simulink model "Ctrl_For_HRV_20260625"  (R2024b)
settings: Solver=ode4  StartTime=0.0  StopTime=22  FixedStep=0.02  RelTol=1e-3
InitFcn:
  | Parameter;
undefined symbols (not defined in the file or in its folder): CCI_DUI_AngleRate_Controller, CCI_DUI_FlowAngle_Controller, fhan, h_alpha, h_beta, h_miu, h_p, h_q, h_r, PNG_2026_6_23, r_alpha, r_beta, r_miu, r_p, r_q, r_r, xishu, xishu_D_0, xishu_L_0, xishu_l_0, xishu_m_0, xishu_n_0, xishu_Y_0
libraries: simulink x60
(part 4 of 8)

== system Ctrl_For_HRV_20260625/Vehicle_2/Error_Model/TD_alpha3 ==
  note: z12
  note: z11
  e_wd_3 : Inport
  Add2 : Sum  Inputs=+-
  Constant : Constant  Value=r_alpha
  Constant1 : Constant  Value=h_alpha
  Integrator : Integrator
  Integrator1 : Integrator
  MATLAB Fcn1 : MATLABFcn  MATLABFcn=fhan(u(1),u(2),u(3),u(4))
  Mux : Mux
  dot_e_wd_3 : Outport  VectorParamsAs1DForOutWhenUnconnected=off
  wires:
  e_wd_3/1 -> Add2/2
  Add2/1 -> Mux/1
  Constant1/1 -> Mux/4
  Constant/1 -> Mux/3
  Mux/1 -> MATLAB Fcn1/1
  MATLAB Fcn1/1 -> Integrator/1
  Integrator1/1 -> Add2/1
  Integrator/1 -> Mux/2, dot_e_wd_3/1, Integrator1/1

== system Ctrl_For_HRV_20260625/Vehicle_2/FlowAngle_Controller_v2/TD_alpha ==
  note: z12
  note: z11
  alpha_d : Inport
  Add2 : Sum  Inputs=+-
  Constant : Constant  Value=r_alpha
  Constant1 : Constant  Value=h_alpha
  Integrator : Integrator
  Integrator1 : Integrator
  MATLAB Fcn1 : MATLABFcn  MATLABFcn=fhan(u(1),u(2),u(3),u(4))
  Mux : Mux
  Scope : Scope
  alpha_c : Outport  VectorParamsAs1DForOutWhenUnconnected=off
  alpha_c_dot : Outport  Port=2  VectorParamsAs1DForOutWhenUnconnected=off
  wires:
  alpha_d/1 -> Add2/2
  Add2/1 -> Mux/1
  Constant1/1 -> Mux/4
  Constant/1 -> Mux/3
  Mux/1 -> MATLAB Fcn1/1
  MATLAB Fcn1/1 -> Integrator/1
  Integrator1/1 -> alpha_c/1, Scope/1, Add2/1
  Integrator/1 -> Mux/2, alpha_c_dot/1, Integrator1/1

== system Ctrl_For_HRV_20260625/Vehicle_2/FlowAngle_Controller_v2/TD_alpha2 ==
  alpha_d : Inport
  Gain17 : Gain  Gain=1.2
  Integrator : Integrator
  Sum : Sum  Inputs=|+-
  alpha_c : Outport
  alpha_c_dot : Outport  Port=2
  wires:
  alpha_d/1 -> Sum/1
  Sum/1 -> Gain17/1
  Integrator/1 -> Sum/2, alpha_c/1
  Gain17/1 -> Integrator/1, alpha_c_dot/1

== system Ctrl_For_HRV_20260625/Vehicle_2/FlowAngle_Controller_v2/TD_alpha3 ==
  note: z12
  note: z11
  dot_beta_c : Inport
  Add2 : Sum  Inputs=+-
  Constant : Constant  Value=r_alpha
  Constant1 : Constant  Value=h_alpha
  Integrator : Integrator
  Integrator1 : Integrator
  MATLAB Fcn1 : MATLABFcn  MATLABFcn=fhan(u(1),u(2),u(3),u(4))
  Mux : Mux
  ddot_beta_c : Outport  VectorParamsAs1DForOutWhenUnconnected=off
  wires:
  dot_beta_c/1 -> Add2/2
  Add2/1 -> Mux/1
  Constant1/1 -> Mux/4
  Constant/1 -> Mux/3
  Mux/1 -> MATLAB Fcn1/1
  MATLAB Fcn1/1 -> Integrator/1
  Integrator1/1 -> Add2/1
  Integrator/1 -> Mux/2, ddot_beta_c/1, Integrator1/1

== system Ctrl_For_HRV_20260625/Vehicle_2/FlowAngle_Controller_v2/TD_alpha4 ==
  note: z12
  note: z11
  dot_miu_c : Inport
  Add2 : Sum  Inputs=+-
  Constant : Constant  Value=r_alpha
  Constant1 : Constant  Value=h_alpha
  Integrator : Integrator
  Integrator1 : Integrator
  MATLAB Fcn1 : MATLABFcn  MATLABFcn=fhan(u(1),u(2),u(3),u(4))
  Mux : Mux
  ddot_miu_c : Outport  VectorParamsAs1DForOutWhenUnconnected=off
  wires:
  dot_miu_c/1 -> Add2/2
  Add2/1 -> Mux/1
  Constant1/1 -> Mux/4
  Constant/1 -> Mux/3
  Mux/1 -> MATLAB Fcn1/1
  MATLAB Fcn1/1 -> Integrator/1
  Integrator1/1 -> Add2/1
  Integrator/1 -> Mux/2, ddot_miu_c/1, Integrator1/1

== system Ctrl_For_HRV_20260625/Vehicle_2/FlowAngle_Controller_v2/TD_beta ==
  note: z12
  note: z11
  beta_d : Inport
  Add2 : Sum  Inputs=+-
  Constant : Constant  Value=r_beta
  Constant1 : Constant  Value=h_beta
  Integrator : Integrator
  Integrator1 : Integrator
  MATLAB Fcn1 : MATLABFcn  MATLABFcn=fhan(u(1),u(2),u(3),u(4))
  Mux : Mux
  beta_c : Outport  VectorParamsAs1DForOutWhenUnconnected=off
  beta_c_dot : Outport  Port=2  VectorParamsAs1DForOutWhenUnconnected=off
  wires:
  beta_d/1 -> Add2/2
  Add2/1 -> Mux/1
  Constant1/1 -> Mux/4
  Constant/1 -> Mux/3
  Mux/1 -> MATLAB Fcn1/1
  MATLAB Fcn1/1 -> Integrator/1
  Integrator1/1 -> beta_c/1, Add2/1
  Integrator/1 -> Mux/2, beta_c_dot/1, Integrator1/1

== system Ctrl_For_HRV_20260625/Vehicle_2/FlowAngle_Controller_v2/TD_beta1 ==
  miu_d : Inport
  Gain17 : Gain  Gain=0.8
  Integrator : Integrator
  Sum : Sum  Inputs=|+-
  miu_c : Outport
  miu_c_dot : Outport  Port=2
  wires:
  miu_d/1 -> Sum/1
  Sum/1 -> Gain17/1
  Integrator/1 -> Sum/2, miu_c/1
  Gain17/1 -> Integrator/1, miu_c_dot/1

== system Ctrl_For_HRV_20260625/Vehicle_2/FlowAngle_Controller_v2/TD_beta2 ==
  beta_d : Inport
  Gain17 : Gain  Gain=1.2
  Integrator : Integrator
  Sum : Sum  Inputs=|+-
  beta_c : Outport
  beta_c_dot : Outport  Port=2
  wires:
  Gain17/1 -> beta_c_dot/1, Integrator/1
  Integrator/1 -> beta_c/1, Sum/2
  Sum/1 -> Gain17/1
  beta_d/1 -> Sum/1

== system Ctrl_For_HRV_20260625/Vehicle_2/FlowAngle_Controller_v2/TD_dotalpha1 ==
  note: z12
  note: z11
  dot_alpha_c : Inport
  Add2 : Sum  Inputs=+-
  Constant : Constant  Value=r_alpha
  Constant1 : Constant  Value=h_alpha
  Integrator : Integrator
  Integrator1 : Integrator
  MATLAB Fcn1 : MATLABFcn  MATLABFcn=fhan(u(1),u(2),u(3),u(4))
  Mux : Mux
  ddot_alpha_c : Outport  VectorParamsAs1DForOutWhenUnconnected=off
  wires:
  dot_alpha_c/1 -> Add2/2
  Add2/1 -> Mux/1
  Constant1/1 -> Mux/4
  Constant/1 -> Mux/3
  Mux/1 -> MATLAB Fcn1/1
  MATLAB Fcn1/1 -> Integrator/1
  Integrator1/1 -> Add2/1
  Integrator/1 -> Mux/2, ddot_alpha_c/1, Integrator1/1

== system Ctrl_For_HRV_20260625/Vehicle_2/FlowAngle_Controller_v2/TD_miu ==
  note: z12
  note: z11
  miu_d : Inport
  Add2 : Sum  Inputs=+-
  Constant : Constant  Value=r_miu
  Constant1 : Constant  Value=h_miu
  Integrator : Integrator
  Integrator1 : Integrator
  MATLAB Fcn1 : MATLABFcn  MATLABFcn=fhan(u(1),u(2),u(3),u(4))
  Mux : Mux
  miu_c : Outport  VectorParamsAs1DForOutWhenUnconnected=off
  miu_c_dot : Outport  Port=2  VectorParamsAs1DForOutWhenUnconnected=off
  wires:
  miu_d/1 -> Add2/2
  Add2/1 -> Mux/1
  Constant1/1 -> Mux/4
  Constant/1 -> Mux/3
  Mux/1 -> MATLAB Fcn1/1
  MATLAB Fcn1/1 -> Integrator/1
  Integrator1/1 -> miu_c/1, Add2/1
  Integrator/1 -> Mux/2, miu_c_dot/1, Integrator1/1

== system Ctrl_For_HRV_20260625/Vehicle_2/HRV_Model_v2/Aerodynamic Parameter perturbation ==
  Band-Limited White Noise : simulink/Sources/Band-Limited White Noise  Cov=1e-6  Ts=2  seed=101
  Band-Limited White Noise1 : simulink/Sources/Band-Limited White Noise  Cov=1e-6  Ts=2  seed=102
  Band-Limited White Noise10 : simulink/Sources/Band-Limited White Noise  Cov=1e-10  Ts=2  seed=103
  Band-Limited White Noise11 : simulink/Sources/Band-Limited White Noise  Cov=1e-10  Ts=2  seed=104
  Band-Limited White Noise12 : simulink/Sources/Band-Limited White Noise  Cov=1e-10  Ts=2  seed=105
  Band-Limited White Noise13 : simulink/Sources/Band-Limited White Noise  Cov=1e-10  Ts=2  seed=106
  Band-Limited White Noise4 : simulink/Sources/Band-Limited White Noise  Cov=1e-6  Ts=2  seed=107
  Band-Limited White Noise5 : simulink/Sources/Band-Limited White Noise  Cov=1e-6  Ts=2  seed=108
  Band-Limited White Noise6 : simulink/Sources/Band-Limited White Noise  Cov=1e-6  Ts=2  seed=109
  Band-Limited White Noise7 : simulink/Sources/Band-Limited White Noise  Cov=1e-6  Ts=2  seed=110
  Band-Limited White Noise8 : simulink/Sources/Band-Limited White Noise  Cov=1e-10  Ts=2  seed=111
  Band-Limited White Noise9 : simulink/Sources/Band-Limited White Noise  Cov=1e-10  Ts=2  seed=112
  Demux : Demux  Outputs=12
  Integrator : Integrator  InitialCondition=[xishu_L_0,xishu_D_0,xishu_Y_0,xishu_l_0,xishu_m_0,xishu_n_0,0,0,0,0,0,0]
  MATLAB Function : MATLAB Function  TreatAsAtomicUnit=on
  Mux : Mux  Inputs=12
  Scope{1..6} (6 alike) : Scope
  To Workspace : ToWorkspace  VariableName=C_L_d_v2  SampleTime=-1
      settings: Save2DSignal=2-D array (concatenate along first dimension)
  To Workspace1 : ToWorkspace  VariableName=C_D_d_v2  SampleTime=-1
      settings: Save2DSignal=2-D array (concatenate along first dimension)
  To Workspace2 : ToWorkspace  VariableName=C_Y_d_v2  SampleTime=-1
      settings: Save2DSignal=2-D array (concatenate along first dimension)
  To Workspace3 : ToWorkspace  VariableName=C_l_d_v2  SampleTime=-1
      settings: Save2DSignal=2-D array (concatenate along first dimension)
  To Workspace4 : ToWorkspace  VariableName=C_m_d_v2  SampleTime=-1
      settings: Save2DSignal=2-D array (concatenate along first dimension)
  To Workspace5 : ToWorkspace  VariableName=C_n_d_v2  SampleTime=-1
      settings: Save2DSignal=2-D array (concatenate along first dimension)
  tag scope: C_D_d_v2=global, C_L_d_v2=global, C_Y_d_v2=global, C_l_d_v2=global, C_m_d_v2=global, C_n_d_v2=global
  wires:
  [C_n_d_v2] -> To Workspace5/1
  [C_m_d_v2] -> To Workspace4/1
  [C_l_d_v2] -> To Workspace3/1
  [C_Y_d_v2] -> To Workspace2/1
  [C_L_d_v2] -> To Workspace/1
  [C_D_d_v2] -> To Workspace1/1
  [C_D_d_v2] -> Scope1/1
  [C_L_d_v2] -> Scope6/1
  [C_l_d_v2] -> Scope3/1
  [C_n_d_v2] -> Scope5/1
  [C_m_d_v2] -> Scope4/1
  [C_Y_d_v2] -> Scope2/1
  Demux/6 -> [C_n_d_v2]
  Demux/5 -> [C_m_d_v2]
  Demux/4 -> [C_l_d_v2]
  Demux/3 -> [C_Y_d_v2]
  Demux/2 -> [C_D_d_v2]
  Demux/1 -> [C_L_d_v2]
  Integrator/1 -> MATLAB Function/1(state), Demux/1
  MATLAB Function/1(dot_state) -> Integrator/1
  Band-Limited White Noise13/1 -> Mux/12
  Band-Limited White Noise12/1 -> Mux/11
  Band-Limited White Noise11/1 -> Mux/10
  Band-Limited White Noise10/1 -> Mux/9
  Band-Limited White Noise9/1 -> Mux/8
  Band-Limited White Noise8/1 -> Mux/7
  Band-Limited White Noise7/1 -> Mux/6
  Band-Limited White Noise6/1 -> Mux/5
  Band-Limited White Noise4/1 -> Mux/3
  Band-Limited White Noise5/1 -> Mux/4
  Band-Limited White Noise1/1 -> Mux/2
  Band-Limited White Noise/1 -> Mux/1
  Mux/1 -> MATLAB Function/2(u)

== system Ctrl_For_HRV_20260625/Vehicle_3/AngleRate_Controller_v3/TD_p ==
  note: z12
  note: z11
  p_d : Inport
  Add2 : Sum  Inputs=+-
  Constant : Constant  Value=r_p
  Constant1 : Constant  Value=h_p
  Integrator : Integrator
  Integrator1 : Integrator
  MATLAB Fcn1 : MATLABFcn  MATLABFcn=fhan(u(1),u(2),u(3),u(4))
  Mux : Mux
  p_c : Outport  VectorParamsAs1DForOutWhenUnconnected=off
  p_c_dot : Outport  Port=2  VectorParamsAs1DForOutWhenUnconnected=off
  wires:
  p_d/1 -> Add2/2
  Add2/1 -> Mux/1
  Constant1/1 -> Mux/4
  Constant/1 -> Mux/3
  Mux/1 -> MATLAB Fcn1/1
  MATLAB Fcn1/1 -> Integrator/1
  Integrator1/1 -> p_c/1, Add2/1
  Integrator/1 -> Mux/2, p_c_dot/1, Integrator1/1

== system Ctrl_For_HRV_20260625/Vehicle_3/AngleRate_Controller_v3/TD_q ==
  note: z12
  note: z11
  q_d : Inport
  Add2 : Sum  Inputs=+-
  Constant : Constant  Value=r_q
  Constant1 : Constant  Value=h_q
  Integrator : Integrator
  Integrator1 : Integrator
  MATLAB Fcn1 : MATLABFcn  MATLABFcn=fhan(u(1),u(2),u(3),u(4))
  Mux : Mux
  q_c : Outport  VectorParamsAs1DForOutWhenUnconnected=off
  q_c_dot : Outport  Port=2  VectorParamsAs1DForOutWhenUnconnected=off
  wires:
  q_d/1 -> Add2/2
  Add2/1 -> Mux/1
  Constant1/1 -> Mux/4
  Constant/1 -> Mux/3
  Mux/1 -> MATLAB Fcn1/1
  MATLAB Fcn1/1 -> Integrator/1
  Integrator1/1 -> q_c/1, Add2/1
  Integrator/1 -> Mux/2, q_c_dot/1, Integrator1/1

== system Ctrl_For_HRV_20260625/Vehicle_3/AngleRate_Controller_v3/TD_r ==
  note: z12
  note: z11
  r_d : Inport
  Add2 : Sum  Inputs=+-
  Constant : Constant  Value=r_r
  Constant1 : Constant  Value=h_r
  Integrator : Integrator
  Integrator1 : Integrator
  MATLAB Fcn1 : MATLABFcn  MATLABFcn=fhan(u(1),u(2),u(3),u(4))
  Mux : Mux
  r_c : Outport  VectorParamsAs1DForOutWhenUnconnected=off
  r_c_dot : Outport  Port=2  VectorParamsAs1DForOutWhenUnconnected=off
  wires:
  r_d/1 -> Add2/2
  Add2/1 -> Mux/1
  Constant1/1 -> Mux/4
  Constant/1 -> Mux/3
  Mux/1 -> MATLAB Fcn1/1
  MATLAB Fcn1/1 -> Integrator/1
  Integrator1/1 -> r_c/1, Add2/1
  Integrator/1 -> Mux/2, r_c_dot/1, Integrator1/1

== system Ctrl_For_HRV_20260625/Vehicle_3/Error_Model/TD_alpha1 ==
  note: z12
  note: z11
  e_wd_1 : Inport
  Add2 : Sum  Inputs=+-
  Constant : Constant  Value=r_alpha
  Constant1 : Constant  Value=h_alpha
  Integrator : Integrator
  Integrator1 : Integrator
  MATLAB Fcn1 : MATLABFcn  MATLABFcn=fhan(u(1),u(2),u(3),u(4))
  Mux : Mux
  dot_e_wd_1 : Outport  VectorParamsAs1DForOutWhenUnconnected=off
  wires:
  e_wd_1/1 -> Add2/2
  Add2/1 -> Mux/1
  Constant1/1 -> Mux/4
  Constant/1 -> Mux/3
  Mux/1 -> MATLAB Fcn1/1
  MATLAB Fcn1/1 -> Integrator/1
  Integrator1/1 -> Add2/1
  Integrator/1 -> Mux/2, dot_e_wd_1/1, Integrator1/1

== system Ctrl_For_HRV_20260625/Vehicle_3/Error_Model/TD_alpha2 ==
  note: z11
  note: z12
  e_wd_2 : Inport
  Add2 : Sum  Inputs=+-
  Constant : Constant  Value=r_alpha
  Constant1 : Constant  Value=h_alpha
  Integrator : Integrator
  Integrator1 : Integrator
  MATLAB Fcn1 : MATLABFcn  MATLABFcn=fhan(u(1),u(2),u(3),u(4))
  Mux : Mux
  dot_e_wd_2 : Outport  VectorParamsAs1DForOutWhenUnconnected=off
  wires:
  Integrator/1 -> Integrator1/1, dot_e_wd_2/1, Mux/2
  Integrator1/1 -> Add2/1
  MATLAB Fcn1/1 -> Integrator/1
  Mux/1 -> MATLAB Fcn1/1
  Constant/1 -> Mux/3
  Constant1/1 -> Mux/4
  Add2/1 -> Mux/1
  e_wd_2/1 -> Add2/2

== system Ctrl_For_HRV_20260625/Vehicle_3/Error_Model/TD_alpha3 ==
  note: z12
  note: z11
  e_wd_3 : Inport
  Add2 : Sum  Inputs=+-
  Constant : Constant  Value=r_alpha
  Constant1 : Constant  Value=h_alpha
  Integrator : Integrator
  Integrator1 : Integrator
  MATLAB Fcn1 : MATLABFcn  MATLABFcn=fhan(u(1),u(2),u(3),u(4))
  Mux : Mux
  dot_e_wd_3 : Outport  VectorParamsAs1DForOutWhenUnconnected=off
  wires:
  e_wd_3/1 -> Add2/2
  Add2/1 -> Mux/1
  Constant1/1 -> Mux/4
  Constant/1 -> Mux/3
  Mux/1 -> MATLAB Fcn1/1
  MATLAB Fcn1/1 -> Integrator/1
  Integrator1/1 -> Add2/1
  Integrator/1 -> Mux/2, dot_e_wd_3/1, Integrator1/1

== system Ctrl_For_HRV_20260625/Vehicle_3/FlowAngle_Controller_v3/TD_alpha ==
  note: z12
  note: z11
  alpha_d : Inport
  Add2 : Sum  Inputs=+-
  Constant : Constant  Value=r_alpha
  Constant1 : Constant  Value=h_alpha
  Integrator : Integrator
  Integrator1 : Integrator
  MATLAB Fcn1 : MATLABFcn  MATLABFcn=fhan(u(1),u(2),u(3),u(4))
  Mux : Mux
  Scope : Scope
  alpha_c : Outport  VectorParamsAs1DForOutWhenUnconnected=off
  alpha_c_dot : Outport  Port=2  VectorParamsAs1DForOutWhenUnconnected=off
  wires:
  alpha_d/1 -> Add2/2
  Add2/1 -> Mux/1
  Constant1/1 -> Mux/4
  Constant/1 -> Mux/3
  Mux/1 -> MATLAB Fcn1/1
  MATLAB Fcn1/1 -> Integrator/1
  Integrator1/1 -> alpha_c/1, Scope/1, Add2/1
  Integrator/1 -> Mux/2, alpha_c_dot/1, Integrator1/1

== system Ctrl_For_HRV_20260625/Vehicle_3/FlowAngle_Controller_v3/TD_alpha2 ==
  alpha_d : Inport
  Gain17 : Gain  Gain=1.2
  Integrator : Integrator
  Sum : Sum  Inputs=|+-
  alpha_c : Outport
  alpha_c_dot : Outport  Port=2
  wires:
  alpha_d/1 -> Sum/1
  Sum/1 -> Gain17/1
  Integrator/1 -> Sum/2, alpha_c/1
  Gain17/1 -> Integrator/1, alpha_c_dot/1

== system Ctrl_For_HRV_20260625/Vehicle_3/FlowAngle_Controller_v3/TD_alpha3 ==
  note: z12
  note: z11
  dot_beta_c : Inport
  Add2 : Sum  Inputs=+-
  Constant : Constant  Value=r_alpha
  Constant1 : Constant  Value=h_alpha
  Integrator : Integrator
  Integrator1 : Integrator
  MATLAB Fcn1 : MATLABFcn  MATLABFcn=fhan(u(1),u(2),u(3),u(4))
  Mux : Mux
  ddot_beta_c : Outport  VectorParamsAs1DForOutWhenUnconnected=off
  wires:
  dot_beta_c/1 -> Add2/2
  Add2/1 -> Mux/1
  Constant1/1 -> Mux/4
  Constant/1 -> Mux/3
  Mux/1 -> MATLAB Fcn1/1
  MATLAB Fcn1/1 -> Integrator/1
  Integrator1/1 -> Add2/1
  Integrator/1 -> Mux/2, ddot_beta_c/1, Integrator1/1

== system Ctrl_For_HRV_20260625/Vehicle_3/FlowAngle_Controller_v3/TD_alpha4 ==
  note: z12
  note: z11
  dot_miu_c : Inport
  Add2 : Sum  Inputs=+-
  Constant : Constant  Value=r_alpha
  Constant1 : Constant  Value=h_alpha
  Integrator : Integrator
  Integrator1 : Integrator
  MATLAB Fcn1 : MATLABFcn  MATLABFcn=fhan(u(1),u(2),u(3),u(4))
  Mux : Mux
  ddot_miu_c : Outport  VectorParamsAs1DForOutWhenUnconnected=off
  wires:
  dot_miu_c/1 -> Add2/2
  Add2/1 -> Mux/1
  Constant1/1 -> Mux/4
  Constant/1 -> Mux/3
  Mux/1 -> MATLAB Fcn1/1
  MATLAB Fcn1/1 -> Integrator/1
  Integrator1/1 -> Add2/1
  Integrator/1 -> Mux/2, ddot_miu_c/1, Integrator1/1

== system Ctrl_For_HRV_20260625/Vehicle_3/FlowAngle_Controller_v3/TD_beta ==
  note: z12
  note: z11
  beta_d : Inport
  Add2 : Sum  Inputs=+-
  Constant : Constant  Value=r_beta
  Constant1 : Constant  Value=h_beta
  Integrator : Integrator
  Integrator1 : Integrator
  MATLAB Fcn1 : MATLABFcn  MATLABFcn=fhan(u(1),u(2),u(3),u(4))
  Mux : Mux
  beta_c : Outport  VectorParamsAs1DForOutWhenUnconnected=off
  beta_c_dot : Outport  Port=2  VectorParamsAs1DForOutWhenUnconnected=off
  wires:
  beta_d/1 -> Add2/2
  Add2/1 -> Mux/1
  Constant1/1 -> Mux/4
  Constant/1 -> Mux/3
  Mux/1 -> MATLAB Fcn1/1
  MATLAB Fcn1/1 -> Integrator/1
  Integrator1/1 -> beta_c/1, Add2/1
  Integrator/1 -> Mux/2, beta_c_dot/1, Integrator1/1

== system Ctrl_For_HRV_20260625/Vehicle_3/FlowAngle_Controller_v3/TD_beta1 ==
  miu_d : Inport
  Gain17 : Gain  Gain=0.8
  Integrator : Integrator
  Sum : Sum  Inputs=|+-
  miu_c : Outport
  miu_c_dot : Outport  Port=2
  wires:
  miu_d/1 -> Sum/1
  Sum/1 -> Gain17/1
  Integrator/1 -> Sum/2, miu_c/1
  Gain17/1 -> Integrator/1, miu_c_dot/1

== system Ctrl_For_HRV_20260625/Vehicle_3/FlowAngle_Controller_v3/TD_beta2 ==
  beta_d : Inport
  Gain17 : Gain  Gain=1.2
  Integrator : Integrator
  Sum : Sum  Inputs=|+-
  beta_c : Outport
  beta_c_dot : Outport  Port=2
  wires:
  Gain17/1 -> beta_c_dot/1, Integrator/1
  Integrator/1 -> beta_c/1, Sum/2
  Sum/1 -> Gain17/1
  beta_d/1 -> Sum/1

== system Ctrl_For_HRV_20260625/Vehicle_3/FlowAngle_Controller_v3/TD_dotalpha1 ==
  note: z12
  note: z11
  dot_alpha_c : Inport
  Add2 : Sum  Inputs=+-
  Constant : Constant  Value=r_alpha
  Constant1 : Constant  Value=h_alpha
  Integrator : Integrator
  Integrator1 : Integrator
  MATLAB Fcn1 : MATLABFcn  MATLABFcn=fhan(u(1),u(2),u(3),u(4))
  Mux : Mux
  ddot_alpha_c : Outport  VectorParamsAs1DForOutWhenUnconnected=off
  wires:
  dot_alpha_c/1 -> Add2/2
  Add2/1 -> Mux/1
  Constant1/1 -> Mux/4
  Constant/1 -> Mux/3
  Mux/1 -> MATLAB Fcn1/1
  MATLAB Fcn1/1 -> Integrator/1
  Integrator1/1 -> Add2/1
  Integrator/1 -> Mux/2, ddot_alpha_c/1, Integrator1/1

== system Ctrl_For_HRV_20260625/Vehicle_3/FlowAngle_Controller_v3/TD_miu ==
  note: z12
  note: z11
  miu_d : Inport
  Add2 : Sum  Inputs=+-
  Constant : Constant  Value=r_miu
  Constant1 : Constant  Value=h_miu
  Integrator : Integrator
  Integrator1 : Integrator
  MATLAB Fcn1 : MATLABFcn  MATLABFcn=fhan(u(1),u(2),u(3),u(4))
  Mux : Mux
  miu_c : Outport  VectorParamsAs1DForOutWhenUnconnected=off
  miu_c_dot : Outport  Port=2  VectorParamsAs1DForOutWhenUnconnected=off
  wires:
  miu_d/1 -> Add2/2
  Add2/1 -> Mux/1
  Constant1/1 -> Mux/4
  Constant/1 -> Mux/3
  Mux/1 -> MATLAB Fcn1/1
  MATLAB Fcn1/1 -> Integrator/1
  Integrator1/1 -> miu_c/1, Add2/1
  Integrator/1 -> Mux/2, miu_c_dot/1, Integrator1/1

== system Ctrl_For_HRV_20260625/Vehicle_3/HRV_Model_v3/Aerodynamic Parameter perturbation ==
  Band-Limited White Noise : simulink/Sources/Band-Limited White Noise  Cov=1e-6  Ts=2  seed=101
  Band-Limited White Noise1 : simulink/Sources/Band-Limited White Noise  Cov=1e-6  Ts=2  seed=102
  Band-Limited White Noise10 : simulink/Sources/Band-Limited White Noise  Cov=1e-10  Ts=2  seed=103
  Band-Limited White Noise11 : simulink/Sources/Band-Limited White Noise  Cov=1e-10  Ts=2  seed=104
  Band-Limited White Noise12 : simulink/Sources/Band-Limited White Noise  Cov=1e-10  Ts=2  seed=105
  Band-Limited White Noise13 : simulink/Sources/Band-Limited White Noise  Cov=1e-10  Ts=2  seed=106
  Band-Limited White Noise4 : simulink/Sources/Band-Limited White Noise  Cov=1e-6  Ts=2  seed=107
  Band-Limited White Noise5 : simulink/Sources/Band-Limited White Noise  Cov=1e-6  Ts=2  seed=108
  Band-Limited White Noise6 : simulink/Sources/Band-Limited White Noise  Cov=1e-6  Ts=2  seed=109
  Band-Limited White Noise7 : simulink/Sources/Band-Limited White Noise  Cov=1e-6  Ts=2  seed=110
  Band-Limited White Noise8 : simulink/Sources/Band-Limited White Noise  Cov=1e-10  Ts=2  seed=111
  Band-Limited White Noise9 : simulink/Sources/Band-Limited White Noise  Cov=1e-10  Ts=2  seed=112
  Demux : Demux  Outputs=12
  Integrator : Integrator  InitialCondition=[xishu_L_0,xishu_D_0,xishu_Y_0,xishu_l_0,xishu_m_0,xishu_n_0,0,0,0,0,0,0]
  MATLAB Function : MATLAB Function  TreatAsAtomicUnit=on
  Mux : Mux  Inputs=12
  Scope{1..6} (6 alike) : Scope
  To Workspace : ToWorkspace  VariableName=C_L_d_v3  SampleTime=-1
      settings: Save2DSignal=2-D array (concatenate along first dimension)
  To Workspace1 : ToWorkspace  VariableName=C_D_d_v3  SampleTime=-1
      settings: Save2DSignal=2-D array (concatenate along first dimension)
  To Workspace2 : ToWorkspace  VariableName=C_Y_d_v3  SampleTime=-1
      settings: Save2DSignal=2-D array (concatenate along first dimension)
  To Workspace3 : ToWorkspace  VariableName=C_l_d_v3  SampleTime=-1
      settings: Save2DSignal=2-D array (concatenate along first dimension)
  To Workspace4 : ToWorkspace  VariableName=C_m_d_v3  SampleTime=-1
      settings: Save2DSignal=2-D array (concatenate along first dimension)
  To Workspace5 : ToWorkspace  VariableName=C_n_d_v3  SampleTime=-1
      settings: Save2DSignal=2-D array (concatenate along first dimension)
  tag scope: C_D_d_v3=global, C_L_d_v3=global, C_Y_d_v3=global, C_l_d_v3=global, C_m_d_v3=global, C_n_d_v3=global
  wires:
  [C_n_d_v3] -> To Workspace5/1
  [C_m_d_v3] -> To Workspace4/1
  [C_l_d_v3] -> To Workspace3/1
  [C_Y_d_v3] -> To Workspace2/1
  [C_L_d_v3] -> To Workspace/1
  [C_D_d_v3] -> To Workspace1/1
  [C_D_d_v3] -> Scope1/1
  [C_L_d_v3] -> Scope6/1
  [C_l_d_v3] -> Scope3/1
  [C_n_d_v3] -> Scope5/1
  [C_m_d_v3] -> Scope4/1
  [C_Y_d_v3] -> Scope2/1
  Demux/6 -> [C_n_d_v3]
  Demux/5 -> [C_m_d_v3]
  Demux/4 -> [C_l_d_v3]
  Demux/3 -> [C_Y_d_v3]
  Demux/2 -> [C_D_d_v3]
  Demux/1 -> [C_L_d_v3]
  Integrator/1 -> MATLAB Function/1(state), Demux/1
  MATLAB Function/1(dot_state) -> Integrator/1
  Band-Limited White Noise13/1 -> Mux/12
  Band-Limited White Noise12/1 -> Mux/11
  Band-Limited White Noise11/1 -> Mux/10
  Band-Limited White Noise10/1 -> Mux/9
  Band-Limited White Noise9/1 -> Mux/8
  Band-Limited White Noise8/1 -> Mux/7
  Band-Limited White Noise7/1 -> Mux/6
  Band-Limited White Noise6/1 -> Mux/5
  Band-Limited White Noise4/1 -> Mux/3
  Band-Limited White Noise5/1 -> Mux/4
  Band-Limited White Noise1/1 -> Mux/2
  Band-Limited White Noise/1 -> Mux/1
  Mux/1 -> MATLAB Function/2(u)

== system Ctrl_For_HRV_20260625/Vehicle_4/AngleRate_Controller_v4/TD_p ==
  note: z12
  note: z11
  p_d : Inport
  Add2 : Sum  Inputs=+-
  Constant : Constant  Value=r_p
  Constant1 : Constant  Value=h_p
  Integrator : Integrator
  Integrator1 : Integrator
  MATLAB Fcn1 : MATLABFcn  MATLABFcn=fhan(u(1),u(2),u(3),u(4))
  Mux : Mux
  p_c : Outport  VectorParamsAs1DForOutWhenUnconnected=off
  p_c_dot : Outport  Port=2  VectorParamsAs1DForOutWhenUnconnected=off
  wires:
  p_d/1 -> Add2/2
  Add2/1 -> Mux/1
  Constant1/1 -> Mux/4
  Constant/1 -> Mux/3
  Mux/1 -> MATLAB Fcn1/1
  MATLAB Fcn1/1 -> Integrator/1
  Integrator1/1 -> p_c/1, Add2/1
  Integrator/1 -> Mux/2, p_c_dot/1, Integrator1/1

== system Ctrl_For_HRV_20260625/Vehicle_4/AngleRate_Controller_v4/TD_q ==
  note: z12
  note: z11
  q_d : Inport
  Add2 : Sum  Inputs=+-
  Constant : Constant  Value=r_q
  Constant1 : Constant  Value=h_q
  Integrator : Integrator
  Integrator1 : Integrator
  MATLAB Fcn1 : MATLABFcn  MATLABFcn=fhan(u(1),u(2),u(3),u(4))
  Mux : Mux
  q_c : Outport  VectorParamsAs1DForOutWhenUnconnected=off
  q_c_dot : Outport  Port=2  VectorParamsAs1DForOutWhenUnconnected=off
  wires:
  q_d/1 -> Add2/2
  Add2/1 -> Mux/1
  Constant1/1 -> Mux/4
  Constant/1 -> Mux/3
  Mux/1 -> MATLAB Fcn1/1
  MATLAB Fcn1/1 -> Integrator/1
  Integrator1/1 -> q_c/1, Add2/1
  Integrator/1 -> Mux/2, q_c_dot/1, Integrator1/1

== system Ctrl_For_HRV_20260625/Vehicle_4/AngleRate_Controller_v4/TD_r ==
  note: z12
  note: z11
  r_d : Inport
  Add2 : Sum  Inputs=+-
  Constant : Constant  Value=r_r
  Constant1 : Constant  Value=h_r
  Integrator : Integrator
  Integrator1 : Integrator
  MATLAB Fcn1 : MATLABFcn  MATLABFcn=fhan(u(1),u(2),u(3),u(4))
  Mux : Mux
  r_c : Outport  VectorParamsAs1DForOutWhenUnconnected=off
  r_c_dot : Outport  Port=2  VectorParamsAs1DForOutWhenUnconnected=off
  wires:
  r_d/1 -> Add2/2
  Add2/1 -> Mux/1
  Constant1/1 -> Mux/4
  Constant/1 -> Mux/3
  Mux/1 -> MATLAB Fcn1/1
  MATLAB Fcn1/1 -> Integrator/1
  Integrator1/1 -> r_c/1, Add2/1
  Integrator/1 -> Mux/2, r_c_dot/1, Integrator1/1

== system Ctrl_For_HRV_20260625/Vehicle_4/Error_Model/TD_alpha1 ==
  note: z12
  note: z11
  e_wd_1 : Inport
  Add2 : Sum  Inputs=+-
  Constant : Constant  Value=r_alpha
  Constant1 : Constant  Value=h_alpha
  Integrator : Integrator
  Integrator1 : Integrator
  MATLAB Fcn1 : MATLABFcn  MATLABFcn=fhan(u(1),u(2),u(3),u(4))
  Mux : Mux
  dot_e_wd_1 : Outport  VectorParamsAs1DForOutWhenUnconnected=off
  wires:
  e_wd_1/1 -> Add2/2
  Add2/1 -> Mux/1
  Constant1/1 -> Mux/4
  Constant/1 -> Mux/3
  Mux/1 -> MATLAB Fcn1/1
  MATLAB Fcn1/1 -> Integrator/1
  Integrator1/1 -> Add2/1
  Integrator/1 -> Mux/2, dot_e_wd_1/1, Integrator1/1

== system Ctrl_For_HRV_20260625/Vehicle_4/Error_Model/TD_alpha2 ==
  note: z11
  note: z12
  e_wd_2 : Inport
  Add2 : Sum  Inputs=+-
  Constant : Constant  Value=r_alpha
  Constant1 : Constant  Value=h_alpha
  Integrator : Integrator
  Integrator1 : Integrator
  MATLAB Fcn1 : MATLABFcn  MATLABFcn=fhan(u(1),u(2),u(3),u(4))
  Mux : Mux
  dot_e_wd_2 : Outport  VectorParamsAs1DForOutWhenUnconnected=off
  wires:
  Integrator/1 -> Integrator1/1, dot_e_wd_2/1, Mux/2
  Integrator1/1 -> Add2/1
  MATLAB Fcn1/1 -> Integrator/1
  Mux/1 -> MATLAB Fcn1/1
  Constant/1 -> Mux/3
  Constant1/1 -> Mux/4
  Add2/1 -> Mux/1
  e_wd_2/1 -> Add2/2

== system Ctrl_For_HRV_20260625/Vehicle_4/Error_Model/TD_alpha3 ==
  note: z12
  note: z11
  e_wd_3 : Inport
  Add2 : Sum  Inputs=+-
  Constant : Constant  Value=r_alpha
  Constant1 : Constant  Value=h_alpha
  Integrator : Integrator
  Integrator1 : Integrator
  MATLAB Fcn1 : MATLABFcn  MATLABFcn=fhan(u(1),u(2),u(3),u(4))
  Mux : Mux
  dot_e_wd_3 : Outport  VectorParamsAs1DForOutWhenUnconnected=off
  wires:
  e_wd_3/1 -> Add2/2
  Add2/1 -> Mux/1
  Constant1/1 -> Mux/4
  Constant/1 -> Mux/3
  Mux/1 -> MATLAB Fcn1/1
  MATLAB Fcn1/1 -> Integrator/1
  Integrator1/1 -> Add2/1
  Integrator/1 -> Mux/2, dot_e_wd_3/1, Integrator1/1

== system Ctrl_For_HRV_20260625/Vehicle_4/FlowAngle_Controller_v4/TD_alpha ==
  note: z12
  note: z11
  alpha_d : Inport
  Add2 : Sum  Inputs=+-
  Constant : Constant  Value=r_alpha
  Constant1 : Constant  Value=h_alpha
  Integrator : Integrator
  Integrator1 : Integrator
  MATLAB Fcn1 : MATLABFcn  MATLABFcn=fhan(u(1),u(2),u(3),u(4))
  Mux : Mux
  Scope : Scope
  alpha_c : Outport  VectorParamsAs1DForOutWhenUnconnected=off
  alpha_c_dot : Outport  Port=2  VectorParamsAs1DForOutWhenUnconnected=off
  wires:
  alpha_d/1 -> Add2/2
  Add2/1 -> Mux/1
  Constant1/1 -> Mux/4
  Constant/1 -> Mux/3
  Mux/1 -> MATLAB Fcn1/1
  MATLAB Fcn1/1 -> Integrator/1
  Integrator1/1 -> alpha_c/1, Scope/1, Add2/1
  Integrator/1 -> Mux/2, alpha_c_dot/1, Integrator1/1

== system Ctrl_For_HRV_20260625/Vehicle_4/FlowAngle_Controller_v4/TD_alpha2 ==
  alpha_d : Inport
  Gain17 : Gain  Gain=1.2
  Integrator : Integrator
  Sum : Sum  Inputs=|+-
  alpha_c : Outport
  alpha_c_dot : Outport  Port=2
  wires:
  alpha_d/1 -> Sum/1
  Sum/1 -> Gain17/1
  Integrator/1 -> Sum/2, alpha_c/1
  Gain17/1 -> Integrator/1, alpha_c_dot/1

== system Ctrl_For_HRV_20260625/Vehicle_4/FlowAngle_Controller_v4/TD_alpha3 ==
  note: z12
  note: z11
  dot_beta_c : Inport
  Add2 : Sum  Inputs=+-
  Constant : Constant  Value=r_alpha
  Constant1 : Constant  Value=h_alpha
  Integrator : Integrator
  Integrator1 : Integrator
  MATLAB Fcn1 : MATLABFcn  MATLABFcn=fhan(u(1),u(2),u(3),u(4))
  Mux : Mux
  ddot_beta_c : Outport  VectorParamsAs1DForOutWhenUnconnected=off
  wires:
  dot_beta_c/1 -> Add2/2
  Add2/1 -> Mux/1
  Constant1/1 -> Mux/4
  Constant/1 -> Mux/3
  Mux/1 -> MATLAB Fcn1/1
  MATLAB Fcn1/1 -> Integrator/1
  Integrator1/1 -> Add2/1
  Integrator/1 -> Mux/2, ddot_beta_c/1, Integrator1/1

== system Ctrl_For_HRV_20260625/Vehicle_4/FlowAngle_Controller_v4/TD_alpha4 ==
  note: z12
  note: z11
  dot_miu_c : Inport
  Add2 : Sum  Inputs=+-
  Constant : Constant  Value=r_alpha
  Constant1 : Constant  Value=h_alpha
  Integrator : Integrator
  Integrator1 : Integrator
  MATLAB Fcn1 : MATLABFcn  MATLABFcn=fhan(u(1),u(2),u(3),u(4))
  Mux : Mux
  ddot_miu_c : Outport  VectorParamsAs1DForOutWhenUnconnected=off
  wires:
  dot_miu_c/1 -> Add2/2
  Add2/1 -> Mux/1
  Constant1/1 -> Mux/4
  Constant/1 -> Mux/3
  Mux/1 -> MATLAB Fcn1/1
  MATLAB Fcn1/1 -> Integrator/1
  Integrator1/1 -> Add2/1
  Integrator/1 -> Mux/2, ddot_miu_c/1, Integrator1/1

== system Ctrl_For_HRV_20260625/Vehicle_4/FlowAngle_Controller_v4/TD_beta ==
  note: z12
  note: z11
  beta_d : Inport
  Add2 : Sum  Inputs=+-
  Constant : Constant  Value=r_beta
  Constant1 : Constant  Value=h_beta
  Integrator : Integrator
  Integrator1 : Integrator
  MATLAB Fcn1 : MATLABFcn  MATLABFcn=fhan(u(1),u(2),u(3),u(4))
  Mux : Mux
  beta_c : Outport  VectorParamsAs1DForOutWhenUnconnected=off
  beta_c_dot : Outport  Port=2  VectorParamsAs1DForOutWhenUnconnected=off
  wires:
  beta_d/1 -> Add2/2
  Add2/1 -> Mux/1
  Constant1/1 -> Mux/4
  Constant/1 -> Mux/3
  Mux/1 -> MATLAB Fcn1/1
  MATLAB Fcn1/1 -> Integrator/1
  Integrator1/1 -> beta_c/1, Add2/1
  Integrator/1 -> Mux/2, beta_c_dot/1, Integrator1/1

== system Ctrl_For_HRV_20260625/Vehicle_4/FlowAngle_Controller_v4/TD_beta1 ==
  miu_d : Inport
  Gain17 : Gain  Gain=0.8
  Integrator : Integrator
  Sum : Sum  Inputs=|+-
  miu_c : Outport
  miu_c_dot : Outport  Port=2
  wires:
  miu_d/1 -> Sum/1
  Sum/1 -> Gain17/1
  Integrator/1 -> Sum/2, miu_c/1
  Gain17/1 -> Integrator/1, miu_c_dot/1

== system Ctrl_For_HRV_20260625/Vehicle_4/FlowAngle_Controller_v4/TD_beta2 ==
  beta_d : Inport
  Gain17 : Gain  Gain=1.2
  Integrator : Integrator
  Sum : Sum  Inputs=|+-
  beta_c : Outport
  beta_c_dot : Outport  Port=2
  wires:
  Gain17/1 -> beta_c_dot/1, Integrator/1
  Integrator/1 -> beta_c/1, Sum/2
  Sum/1 -> Gain17/1
  beta_d/1 -> Sum/1

== system Ctrl_For_HRV_20260625/Vehicle_4/FlowAngle_Controller_v4/TD_dotalpha1 ==
  note: z12
  note: z11
  dot_alpha_c : Inport
  Add2 : Sum  Inputs=+-
  Constant : Constant  Value=r_alpha
  Constant1 : Constant  Value=h_alpha
  Integrator : Integrator
  Integrator1 : Integrator
  MATLAB Fcn1 : MATLABFcn  MATLABFcn=fhan(u(1),u(2),u(3),u(4))
  Mux : Mux
  ddot_alpha_c : Outport  VectorParamsAs1DForOutWhenUnconnected=off
  wires:
  dot_alpha_c/1 -> Add2/2
  Add2/1 -> Mux/1
  Constant1/1 -> Mux/4
  Constant/1 -> Mux/3
  Mux/1 -> MATLAB Fcn1/1
  MATLAB Fcn1/1 -> Integrator/1
  Integrator1/1 -> Add2/1
  Integrator/1 -> Mux/2, ddot_alpha_c/1, Integrator1/1

== system Ctrl_For_HRV_20260625/Vehicle_4/FlowAngle_Controller_v4/TD_miu ==
  note: z12
  note: z11
  miu_d : Inport
  Add2 : Sum  Inputs=+-
  Constant : Constant  Value=r_miu
  Constant1 : Constant  Value=h_miu
  Integrator : Integrator
  Integrator1 : Integrator
  MATLAB Fcn1 : MATLABFcn  MATLABFcn=fhan(u(1),u(2),u(3),u(4))
  Mux : Mux
  miu_c : Outport  VectorParamsAs1DForOutWhenUnconnected=off
  miu_c_dot : Outport  Port=2  VectorParamsAs1DForOutWhenUnconnected=off
  wires:
  miu_d/1 -> Add2/2
  Add2/1 -> Mux/1
  Constant1/1 -> Mux/4
  Constant/1 -> Mux/3
  Mux/1 -> MATLAB Fcn1/1
  MATLAB Fcn1/1 -> Integrator/1
  Integrator1/1 -> miu_c/1, Add2/1
  Integrator/1 -> Mux/2, miu_c_dot/1, Integrator1/1

== system Ctrl_For_HRV_20260625/Vehicle_4/HRV_Model_v4/Aerodynamic Parameter perturbation ==
  Band-Limited White Noise : simulink/Sources/Band-Limited White Noise  Cov=1e-6  Ts=2  seed=101
  Band-Limited White Noise1 : simulink/Sources/Band-Limited White Noise  Cov=1e-6  Ts=2  seed=102
  Band-Limited White Noise10 : simulink/Sources/Band-Limited White Noise  Cov=1e-10  Ts=2  seed=103
  Band-Limited White Noise11 : simulink/Sources/Band-Limited White Noise  Cov=1e-10  Ts=2  seed=104
  Band-Limited White Noise12 : simulink/Sources/Band-Limited White Noise  Cov=1e-10  Ts=2  seed=105
  Band-Limited White Noise13 : simulink/Sources/Band-Limited White Noise  Cov=1e-10  Ts=2  seed=106
  Band-Limited White Noise4 : simulink/Sources/Band-Limited White Noise  Cov=1e-6  Ts=2  seed=107
  Band-Limited White Noise5 : simulink/Sources/Band-Limited White Noise  Cov=1e-6  Ts=2  seed=108
  Band-Limited White Noise6 : simulink/Sources/Band-Limited White Noise  Cov=1e-6  Ts=2  seed=109
  Band-Limited White Noise7 : simulink/Sources/Band-Limited White Noise  Cov=1e-6  Ts=2  seed=110
  Band-Limited White Noise8 : simulink/Sources/Band-Limited White Noise  Cov=1e-10  Ts=2  seed=111
  Band-Limited White Noise9 : simulink/Sources/Band-Limited White Noise  Cov=1e-10  Ts=2  seed=112
  Demux : Demux  Outputs=12
  Integrator : Integrator  InitialCondition=[xishu_L_0,xishu_D_0,xishu_Y_0,xishu_l_0,xishu_m_0,xishu_n_0,0,0,0,0,0,0]
  MATLAB Function : MATLAB Function  TreatAsAtomicUnit=on
  Mux : Mux  Inputs=12
  Scope{1..6} (6 alike) : Scope
  To Workspace : ToWorkspace  VariableName=C_L_d_v4  SampleTime=-1
      settings: Save2DSignal=2-D array (concatenate along first dimension)
  To Workspace1 : ToWorkspace  VariableName=C_D_d_v4  SampleTime=-1
      settings: Save2DSignal=2-D array (concatenate along first dimension)
  To Workspace2 : ToWorkspace  VariableName=C_Y_d_v4  SampleTime=-1
      settings: Save2DSignal=2-D array (concatenate along first dimension)
  To Workspace3 : ToWorkspace  VariableName=C_l_d_v4  SampleTime=-1
      settings: Save2DSignal=2-D array (concatenate along first dimension)
  To Workspace4 : ToWorkspace  VariableName=C_m_d_v4  SampleTime=-1
      settings: Save2DSignal=2-D array (concatenate along first dimension)
  To Workspace5 : ToWorkspace  VariableName=C_n_d_v4  SampleTime=-1
      settings: Save2DSignal=2-D array (concatenate along first dimension)
  tag scope: C_D_d_v4=global, C_L_d_v4=global, C_Y_d_v4=global, C_l_d_v4=global, C_m_d_v4=global, C_n_d_v4=global
  wires:
  [C_n_d_v4] -> To Workspace5/1
  [C_m_d_v4] -> To Workspace4/1
  [C_l_d_v4] -> To Workspace3/1
  [C_Y_d_v4] -> To Workspace2/1
  [C_L_d_v4] -> To Workspace/1
  [C_D_d_v4] -> To Workspace1/1
  [C_D_d_v4] -> Scope1/1
  [C_L_d_v4] -> Scope6/1
  [C_l_d_v4] -> Scope3/1
  [C_n_d_v4] -> Scope5/1
  [C_m_d_v4] -> Scope4/1
  [C_Y_d_v4] -> Scope2/1
  Demux/6 -> [C_n_d_v4]
  Demux/5 -> [C_m_d_v4]
  Demux/4 -> [C_l_d_v4]
  Demux/3 -> [C_Y_d_v4]
  Demux/2 -> [C_D_d_v4]
  Demux/1 -> [C_L_d_v4]
  Integrator/1 -> MATLAB Function/1(state), Demux/1
  MATLAB Function/1(dot_state) -> Integrator/1
  Band-Limited White Noise13/1 -> Mux/12
  Band-Limited White Noise12/1 -> Mux/11
  Band-Limited White Noise11/1 -> Mux/10
  Band-Limited White Noise10/1 -> Mux/9
  Band-Limited White Noise9/1 -> Mux/8
  Band-Limited White Noise8/1 -> Mux/7
  Band-Limited White Noise7/1 -> Mux/6
  Band-Limited White Noise6/1 -> Mux/5
  Band-Limited White Noise4/1 -> Mux/3
  Band-Limited White Noise5/1 -> Mux/4
  Band-Limited White Noise1/1 -> Mux/2
  Band-Limited White Noise/1 -> Mux/1
  Mux/1 -> MATLAB Function/2(u)

== system Ctrl_For_HRV_20260625/Vehicle_5/AngleRate_Controller_v5/TD_p ==
  note: z12
  note: z11
  p_d : Inport
  Add2 : Sum  Inputs=+-
  Constant : Constant  Value=r_p
  Constant1 : Constant  Value=h_p
  Integrator : Integrator
  Integrator1 : Integrator
  MATLAB Fcn1 : MATLABFcn  MATLABFcn=fhan(u(1),u(2),u(3),u(4))
  Mux : Mux
  p_c : Outport  VectorParamsAs1DForOutWhenUnconnected=off
  p_c_dot : Outport  Port=2  VectorParamsAs1DForOutWhenUnconnected=off
  wires:
  p_d/1 -> Add2/2
  Add2/1 -> Mux/1
  Constant1/1 -> Mux/4
  Constant/1 -> Mux/3
  Mux/1 -> MATLAB Fcn1/1
  MATLAB Fcn1/1 -> Integrator/1
  Integrator1/1 -> p_c/1, Add2/1
  Integrator/1 -> Mux/2, p_c_dot/1, Integrator1/1

== system Ctrl_For_HRV_20260625/Vehicle_5/AngleRate_Controller_v5/TD_q ==
  note: z12
  note: z11
  q_d : Inport
  Add2 : Sum  Inputs=+-
  Constant : Constant  Value=r_q
  Constant1 : Constant  Value=h_q
  Integrator : Integrator
  Integrator1 : Integrator
  MATLAB Fcn1 : MATLABFcn  MATLABFcn=fhan(u(1),u(2),u(3),u(4))
  Mux : Mux
  q_c : Outport  VectorParamsAs1DForOutWhenUnconnected=off
  q_c_dot : Outport  Port=2  VectorParamsAs1DForOutWhenUnconnected=off
  wires:
  q_d/1 -> Add2/2
  Add2/1 -> Mux/1
  Constant1/1 -> Mux/4
  Constant/1 -> Mux/3
  Mux/1 -> MATLAB Fcn1/1
  MATLAB Fcn1/1 -> Integrator/1
  Integrator1/1 -> q_c/1, Add2/1
  Integrator/1 -> Mux/2, q_c_dot/1, Integrator1/1

== system Ctrl_For_HRV_20260625/Vehicle_5/AngleRate_Controller_v5/TD_r ==
  note: z12
  note: z11
  r_d : Inport
  Add2 : Sum  Inputs=+-
  Constant : Constant  Value=r_r
  Constant1 : Constant  Value=h_r
  Integrator : Integrator
  Integrator1 : Integrator
  MATLAB Fcn1 : MATLABFcn  MATLABFcn=fhan(u(1),u(2),u(3),u(4))
  Mux : Mux
  r_c : Outport  VectorParamsAs1DForOutWhenUnconnected=off
  r_c_dot : Outport  Port=2  VectorParamsAs1DForOutWhenUnconnected=off
  wires:
  r_d/1 -> Add2/2
  Add2/1 -> Mux/1
  Constant1/1 -> Mux/4
  Constant/1 -> Mux/3
  Mux/1 -> MATLAB Fcn1/1
  MATLAB Fcn1/1 -> Integrator/1
  Integrator1/1 -> r_c/1, Add2/1
  Integrator/1 -> Mux/2, r_c_dot/1, Integrator1/1

== system Ctrl_For_HRV_20260625/Vehicle_5/Error_Model/TD_alpha1 ==
  note: z12
  note: z11
  e_wd_1 : Inport
  Add2 : Sum  Inputs=+-
  Constant : Constant  Value=r_alpha
  Constant1 : Constant  Value=h_alpha
  Integrator : Integrator
  Integrator1 : Integrator
  MATLAB Fcn1 : MATLABFcn  MATLABFcn=fhan(u(1),u(2),u(3),u(4))
  Mux : Mux
  dot_e_wd_1 : Outport  VectorParamsAs1DForOutWhenUnconnected=off
  wires:
  e_wd_1/1 -> Add2/2
  Add2/1 -> Mux/1
  Constant1/1 -> Mux/4
  Constant/1 -> Mux/3
  Mux/1 -> MATLAB Fcn1/1
  MATLAB Fcn1/1 -> Integrator/1
  Integrator1/1 -> Add2/1
  Integrator/1 -> Mux/2, dot_e_wd_1/1, Integrator1/1

== system Ctrl_For_HRV_20260625/Vehicle_5/Error_Model/TD_alpha2 ==
  note: z11
  note: z12
  e_wd_2 : Inport
  Add2 : Sum  Inputs=+-
  Constant : Constant  Value=r_alpha
  Constant1 : Constant  Value=h_alpha
  Integrator : Integrator
  Integrator1 : Integrator
  MATLAB Fcn1 : MATLABFcn  MATLABFcn=fhan(u(1),u(2),u(3),u(4))
  Mux : Mux
  dot_e_wd_2 : Outport  VectorParamsAs1DForOutWhenUnconnected=off
  wires:
  Integrator/1 -> Integrator1/1, dot_e_wd_2/1, Mux/2
  Integrator1/1 -> Add2/1
  MATLAB Fcn1/1 -> Integrator/1
  Mux/1 -> MATLAB Fcn1/1
  Constant/1 -> Mux/3
  Constant1/1 -> Mux/4
  Add2/1 -> Mux/1
  e_wd_2/1 -> Add2/2

== system Ctrl_For_HRV_20260625/Vehicle_5/Error_Model/TD_alpha3 ==
  note: z12
  note: z11
  e_wd_3 : Inport
  Add2 : Sum  Inputs=+-
  Constant : Constant  Value=r_alpha
  Constant1 : Constant  Value=h_alpha
  Integrator : Integrator
  Integrator1 : Integrator
  MATLAB Fcn1 : MATLABFcn  MATLABFcn=fhan(u(1),u(2),u(3),u(4))
  Mux : Mux
  dot_e_wd_3 : Outport  VectorParamsAs1DForOutWhenUnconnected=off
  wires:
  e_wd_3/1 -> Add2/2
  Add2/1 -> Mux/1
  Constant1/1 -> Mux/4
  Constant/1 -> Mux/3
  Mux/1 -> MATLAB Fcn1/1
  MATLAB Fcn1/1 -> Integrator/1
  Integrator1/1 -> Add2/1
  Integrator/1 -> Mux/2, dot_e_wd_3/1, Integrator1/1

== system Ctrl_For_HRV_20260625/Vehicle_5/FlowAngle_Controller_v5/TD_alpha ==
  note: z12
  note: z11
  alpha_d : Inport
  Add2 : Sum  Inputs=+-
  Constant : Constant  Value=r_alpha
  Constant1 : Constant  Value=h_alpha
  Integrator : Integrator
  Integrator1 : Integrator
  MATLAB Fcn1 : MATLABFcn  MATLABFcn=fhan(u(1),u(2),u(3),u(4))
  Mux : Mux
  Scope : Scope
  alpha_c : Outport  VectorParamsAs1DForOutWhenUnconnected=off
  alpha_c_dot : Outport  Port=2  VectorParamsAs1DForOutWhenUnconnected=off
  wires:
  alpha_d/1 -> Add2/2
  Add2/1 -> Mux/1
  Constant1/1 -> Mux/4
  Constant/1 -> Mux/3
  Mux/1 -> MATLAB Fcn1/1
  MATLAB Fcn1/1 -> Integrator/1
  Integrator1/1 -> alpha_c/1, Scope/1, Add2/1
  Integrator/1 -> Mux/2, alpha_c_dot/1, Integrator1/1

== system Ctrl_For_HRV_20260625/Vehicle_5/FlowAngle_Controller_v5/TD_alpha2 ==
  alpha_d : Inport
  Gain17 : Gain  Gain=1.2
  Integrator : Integrator
  Sum : Sum  Inputs=|+-
  alpha_c : Outport
  alpha_c_dot : Outport  Port=2
  wires:
  alpha_d/1 -> Sum/1
  Sum/1 -> Gain17/1
  Integrator/1 -> Sum/2, alpha_c/1
  Gain17/1 -> Integrator/1, alpha_c_dot/1

== system Ctrl_For_HRV_20260625/Vehicle_5/FlowAngle_Controller_v5/TD_alpha3 ==
  note: z12
  note: z11
  dot_beta_c : Inport
  Add2 : Sum  Inputs=+-
  Constant : Constant  Value=r_alpha
  Constant1 : Constant  Value=h_alpha
  Integrator : Integrator
  Integrator1 : Integrator
  MATLAB Fcn1 : MATLABFcn  MATLABFcn=fhan(u(1),u(2),u(3),u(4))
  Mux : Mux
  ddot_beta_c : Outport  VectorParamsAs1DForOutWhenUnconnected=off
  wires:
  dot_beta_c/1 -> Add2/2
  Add2/1 -> Mux/1
  Constant1/1 -> Mux/4
  Constant/1 -> Mux/3
  Mux/1 -> MATLAB Fcn1/1
  MATLAB Fcn1/1 -> Integrator/1
  Integrator1/1 -> Add2/1
  Integrator/1 -> Mux/2, ddot_beta_c/1, Integrator1/1

== system Ctrl_For_HRV_20260625/Vehicle_5/FlowAngle_Controller_v5/TD_alpha4 ==
  note: z12
  note: z11
  dot_miu_c : Inport
  Add2 : Sum  Inputs=+-
  Constant : Constant  Value=r_alpha
  Constant1 : Constant  Value=h_alpha
  Integrator : Integrator
  Integrator1 : Integrator
  MATLAB Fcn1 : MATLABFcn  MATLABFcn=fhan(u(1),u(2),u(3),u(4))
  Mux : Mux
  ddot_miu_c : Outport  VectorParamsAs1DForOutWhenUnconnected=off
  wires:
  dot_miu_c/1 -> Add2/2
  Add2/1 -> Mux/1
  Constant1/1 -> Mux/4
  Constant/1 -> Mux/3
  Mux/1 -> MATLAB Fcn1/1
  MATLAB Fcn1/1 -> Integrator/1
  Integrator1/1 -> Add2/1
  Integrator/1 -> Mux/2, ddot_miu_c/1, Integrator1/1

== system Ctrl_For_HRV_20260625/Vehicle_5/FlowAngle_Controller_v5/TD_beta ==
  note: z12
  note: z11
  beta_d : Inport
  Add2 : Sum  Inputs=+-
  Constant : Constant  Value=r_beta
  Constant1 : Constant  Value=h_beta
  Integrator : Integrator
  Integrator1 : Integrator
  MATLAB Fcn1 : MATLABFcn  MATLABFcn=fhan(u(1),u(2),u(3),u(4))
  Mux : Mux
  beta_c : Outport  VectorParamsAs1DForOutWhenUnconnected=off
  beta_c_dot : Outport  Port=2  VectorParamsAs1DForOutWhenUnconnected=off
  wires:
  beta_d/1 -> Add2/2
  Add2/1 -> Mux/1
  Constant1/1 -> Mux/4
  Constant/1 -> Mux/3
  Mux/1 -> MATLAB Fcn1/1
  MATLAB Fcn1/1 -> Integrator/1
  Integrator1/1 -> beta_c/1, Add2/1
  Integrator/1 -> Mux/2, beta_c_dot/1, Integrator1/1

== system Ctrl_For_HRV_20260625/Vehicle_5/FlowAngle_Controller_v5/TD_beta1 ==
  miu_d : Inport
  Gain17 : Gain  Gain=0.8
  Integrator : Integrator
  Sum : Sum  Inputs=|+-
  miu_c : Outport
  miu_c_dot : Outport  Port=2
  wires:
  miu_d/1 -> Sum/1
  Sum/1 -> Gain17/1
  Integrator/1 -> Sum/2, miu_c/1
  Gain17/1 -> Integrator/1, miu_c_dot/1

== system Ctrl_For_HRV_20260625/Vehicle_5/FlowAngle_Controller_v5/TD_beta2 ==
  beta_d : Inport
  Gain17 : Gain  Gain=1.2
  Integrator : Integrator
  Sum : Sum  Inputs=|+-
  beta_c : Outport
  beta_c_dot : Outport  Port=2
  wires:
  Gain17/1 -> beta_c_dot/1, Integrator/1
  Integrator/1 -> beta_c/1, Sum/2
  Sum/1 -> Gain17/1
  beta_d/1 -> Sum/1

== system Ctrl_For_HRV_20260625/Vehicle_5/FlowAngle_Controller_v5/TD_dotalpha1 ==
  note: z12
  note: z11
  dot_alpha_c : Inport
  Add2 : Sum  Inputs=+-
  Constant : Constant  Value=r_alpha
  Constant1 : Constant  Value=h_alpha
  Integrator : Integrator
  Integrator1 : Integrator
  MATLAB Fcn1 : MATLABFcn  MATLABFcn=fhan(u(1),u(2),u(3),u(4))
  Mux : Mux
  ddot_alpha_c : Outport  VectorParamsAs1DForOutWhenUnconnected=off
  wires:
  dot_alpha_c/1 -> Add2/2
  Add2/1 -> Mux/1
  Constant1/1 -> Mux/4
  Constant/1 -> Mux/3
  Mux/1 -> MATLAB Fcn1/1
  MATLAB Fcn1/1 -> Integrator/1
  Integrator1/1 -> Add2/1
  Integrator/1 -> Mux/2, ddot_alpha_c/1, Integrator1/1

== system Ctrl_For_HRV_20260625/Vehicle_5/FlowAngle_Controller_v5/TD_miu ==
  note: z12
  note: z11
  miu_d : Inport
  Add2 : Sum  Inputs=+-
  Constant : Constant  Value=r_miu
  Constant1 : Constant  Value=h_miu
  Integrator : Integrator
  Integrator1 : Integrator
  MATLAB Fcn1 : MATLABFcn  MATLABFcn=fhan(u(1),u(2),u(3),u(4))
  Mux : Mux
  miu_c : Outport  VectorParamsAs1DForOutWhenUnconnected=off
  miu_c_dot : Outport  Port=2  VectorParamsAs1DForOutWhenUnconnected=off
  wires:
  miu_d/1 -> Add2/2
  Add2/1 -> Mux/1
  Constant1/1 -> Mux/4
  Constant/1 -> Mux/3
  Mux/1 -> MATLAB Fcn1/1
  MATLAB Fcn1/1 -> Integrator/1
  Integrator1/1 -> miu_c/1, Add2/1
  Integrator/1 -> Mux/2, miu_c_dot/1, Integrator1/1

== system Ctrl_For_HRV_20260625/Vehicle_5/HRV_Model_v5/Aerodynamic Parameter perturbation ==
  Band-Limited White Noise : simulink/Sources/Band-Limited White Noise  Cov=1e-6  Ts=2  seed=101
  Band-Limited White Noise1 : simulink/Sources/Band-Limited White Noise  Cov=1e-6  Ts=2  seed=102
  Band-Limited White Noise10 : simulink/Sources/Band-Limited White Noise  Cov=1e-10  Ts=2  seed=103
  Band-Limited White Noise11 : simulink/Sources/Band-Limited White Noise  Cov=1e-10  Ts=2  seed=104
  Band-Limited White Noise12 : simulink/Sources/Band-Limited White Noise  Cov=1e-10  Ts=2  seed=105
  Band-Limited White Noise13 : simulink/Sources/Band-Limited White Noise  Cov=1e-10  Ts=2  seed=106
  Band-Limited White Noise4 : simulink/Sources/Band-Limited White Noise  Cov=1e-6  Ts=2  seed=107
  Band-Limited White Noise5 : simulink/Sources/Band-Limited White Noise  Cov=1e-6  Ts=2  seed=108
  Band-Limited White Noise6 : simulink/Sources/Band-Limited White Noise  Cov=1e-6  Ts=2  seed=109
  Band-Limited White Noise7 : simulink/Sources/Band-Limited White Noise  Cov=1e-6  Ts=2  seed=110
  Band-Limited White Noise8 : simulink/Sources/Band-Limited White Noise  Cov=1e-10  Ts=2  seed=111
  Band-Limited White Noise9 : simulink/Sources/Band-Limited White Noise  Cov=1e-10  Ts=2  seed=112
  Demux : Demux  Outputs=12
  Integrator : Integrator  InitialCondition=[xishu_L_0,xishu_D_0,xishu_Y_0,xishu_l_0,xishu_m_0,xishu_n_0,0,0,0,0,0,0]
  MATLAB Function : MATLAB Function  TreatAsAtomicUnit=on
  Mux : Mux  Inputs=12
  Scope{1..6} (6 alike) : Scope
  To Workspace : ToWorkspace  VariableName=C_L_d_v5  SampleTime=-1
      settings: Save2DSignal=2-D array (concatenate along first dimension)
  To Workspace1 : ToWorkspace  VariableName=C_D_d_v5  SampleTime=-1
      settings: Save2DSignal=2-D array (concatenate along first dimension)
  To Workspace2 : ToWorkspace  VariableName=C_Y_d_v5  SampleTime=-1
      settings: Save2DSignal=2-D array (concatenate along first dimension)
  To Workspace3 : ToWorkspace  VariableName=C_l_d_v5  SampleTime=-1
      settings: Save2DSignal=2-D array (concatenate along first dimension)
  To Workspace4 : ToWorkspace  VariableName=C_m_d_v5  SampleTime=-1
      settings: Save2DSignal=2-D array (concatenate along first dimension)
  To Workspace5 : ToWorkspace  VariableName=C_n_d_v5  SampleTime=-1
      settings: Save2DSignal=2-D array (concatenate along first dimension)
  tag scope: C_D_d_v5=global, C_L_d_v5=global, C_Y_d_v5=global, C_l_d_v5=global, C_m_d_v5=global, C_n_d_v5=global
  wires:
  [C_n_d_v5] -> To Workspace5/1
  [C_m_d_v5] -> To Workspace4/1
  [C_l_d_v5] -> To Workspace3/1
  [C_Y_d_v5] -> To Workspace2/1
  [C_L_d_v5] -> To Workspace/1
  [C_D_d_v5] -> To Workspace1/1
  [C_D_d_v5] -> Scope1/1
  [C_L_d_v5] -> Scope6/1
  [C_l_d_v5] -> Scope3/1
  [C_n_d_v5] -> Scope5/1
  [C_m_d_v5] -> Scope4/1
  [C_Y_d_v5] -> Scope2/1
  Demux/6 -> [C_n_d_v5]
  Demux/5 -> [C_m_d_v5]
  Demux/4 -> [C_l_d_v5]
  Demux/3 -> [C_Y_d_v5]
  Demux/2 -> [C_D_d_v5]
  Demux/1 -> [C_L_d_v5]
  Integrator/1 -> MATLAB Function/1(state), Demux/1
  MATLAB Function/1(dot_state) -> Integrator/1
  Band-Limited White Noise13/1 -> Mux/12
  Band-Limited White Noise12/1 -> Mux/11
  Band-Limited White Noise11/1 -> Mux/10
  Band-Limited White Noise10/1 -> Mux/9
  Band-Limited White Noise9/1 -> Mux/8
  Band-Limited White Noise8/1 -> Mux/7
  Band-Limited White Noise7/1 -> Mux/6
  Band-Limited White Noise6/1 -> Mux/5
  Band-Limited White Noise4/1 -> Mux/3
  Band-Limited White Noise5/1 -> Mux/4
  Band-Limited White Noise1/1 -> Mux/2
  Band-Limited White Noise/1 -> Mux/1
  Mux/1 -> MATLAB Function/2(u)

== matlab function Ctrl_For_HRV_20260625/Vehicle_2/HRV_Model_v2/Aerodynamic Parameter perturbation/MATLAB Function ==
  data: state input; dot_state output; u input
function dot_state  = Shedong_Model(state,u)
    C_L_d = state(1);C_D_d = state(2);C_Y_d = state(3);C_l_d = state(4);C_m_d = state(5);C_n_d = state(6);
    xi_L = state(7);xi_D = state(8);xi_Y = state(9);xi_l = state(10);xi_m = state(11);xi_n = state(12);
    omega_C_L_d = u(1);omega_C_D_d = u(2);omega_C_Y_d = u(3);omega_C_l_d = u(4);omega_C_m_d = u(5);omega_C_n_d = u(6);
    omega_xi_L_d = u(7);omega_xi_D_d = u(8);omega_xi_Y_d = u(9);omega_xi_l_d = u(10);omega_xi_m_d = u(11);omega_xi_n_d = u(12);

    dot_C_L_d = -xi_L*C_L_d+omega_C_L_d;    
    dot_C_D_d = -xi_D*C_D_d+omega_C_D_d;
    dot_C_Y_d = -xi_Y*C_Y_d+omega_C_Y_d;
    dot_C_l_d = -xi_l*C_l_d+omega_C_l_d;
    dot_C_m_d = -xi_m*C_m_d+omega_C_m_d;
    dot_C_n_d = -xi_n*C_n_d+omega_C_n_d;
    dot_xi_L = omega_xi_L_d;
    dot_xi_D = omega_xi_D_d;
    dot_xi_Y = omega_xi_Y_d;
    dot_xi_l = omega_xi_l_d;
    dot_xi_m = omega_xi_m_d;
    dot_xi_n = omega_xi_n_d;
            
    dot_state = [dot_C_L_d,dot_C_D_d,dot_C_Y_d,dot_C_l_d,dot_C_m_d,dot_C_n_d,dot_xi_L,dot_xi_D,dot_xi_Y,dot_xi_l,dot_xi_m,dot_xi_n];
end
